simulink model "luenberger"  (Simulink 8.3)
settings: Solver=ode4  StartTime=0.0  StopTime=10.0  FixedStep=0.01  RelTol=1e-3
values from neighbouring files (symbols this model uses):
  A = [0 1 ... (first row only)    [por_model_obiekt_osX.m]    (also in wykresy.m)
  B = [0; k/omega0^2]    [por_model_obiekt_osX.m]    (also in wykresy.m)
  C = [1 0]    [por_model_obiekt_osX.m]    (also in wykresy.m)
  L = transpose(place(transpose(Al),transpose(Cl), [-1 -0.9 -1.1]))    [luenberger.m]
  X0 = [0 0]    [por_model_obiekt_osX.m]    (also in wykresy.m = [0.2738 0])
undefined symbols (not defined in the file or in its folder): A_, B_, C_
libraries: simulink x1
settings Model: Creator=student  LastModifiedBy=Maciek  CovSFcnEnable=on
settings OptimizationCC: ExpressionDepthLimit=2147483647
settings DebuggingCC: FcnCallInpInsideContextMsg=EnableAllAsWarning  FrameProcessingCompatibilityMsg=error
settings GRTTargetCC: CombineOutputUpdateFcns=on  GRTInterface=off

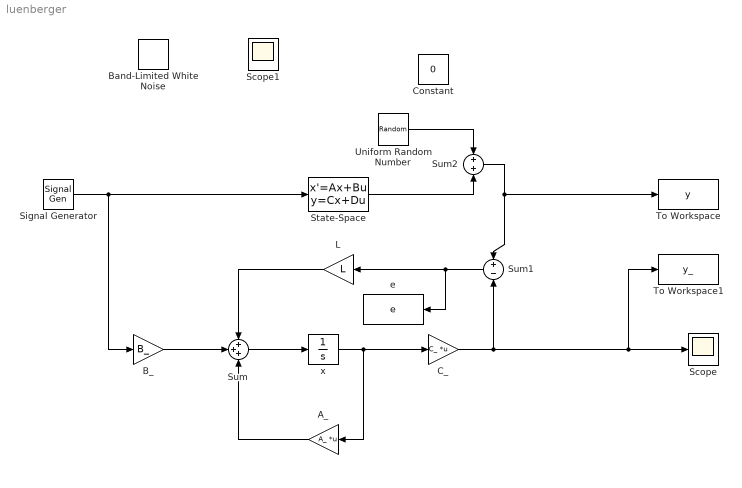
== system luenberger ==
  A_ : Gain  Gain=A_  Multiplication=Matrix(K*u) (u vector)
  B_ : Gain  Gain=B_
  Band-Limited White Noise : simulink/Sources/Band-Limited White Noise  Cov=[0.1]  Ts=0.1  seed=[23341]
  C_ : Gain  Gain=C_  Multiplication=Matrix(K*u) (u vector)
  Constant : Constant  Value=0
  L : Gain  Gain=L
  Scope : Scope
      settings: TimeRange=auto  LimitDataPoints=on  MaxDataPoints=5000  SaveToWorkspace=off  SaveName=ScopeData  YMin=-10  YMax=10  SampleTime=-1
  Scope1 : Scope
      settings: TimeRange=auto  LimitDataPoints=on  MaxDataPoints=5000  SaveToWorkspace=off  YMin=-1.00000  YMax=1.00000  SampleTime=-1
  Signal Generator : SignalGenerator
  State-Space : StateSpace  A=A  B=B  C=C  D=0  X0=X0
  Sum : Sum  Inputs=+++
  Sum1 : Sum  Inputs=+-
  Sum2 : Sum
  To Workspace : ToWorkspace  VariableName=y  SaveFormat=Timeseries  SampleTime=-1
  To Workspace1 : ToWorkspace  VariableName=y_  SaveFormat=Timeseries  SampleTime=-1
  Uniform Random Number : UniformRandomNumber  Minimum=-0.001  Maximum=0.001
  e : ToWorkspace  VariableName=e  SaveFormat=Timeseries  SampleTime=-1
  x : Integrator  InitialCondition=X0
  wires:
  Sum/1 -> x/1
  x/1 -> A_/1, C_/1
  A_/1 -> Sum/3
  C_/1 -> Sum1/2, Scope/1, To Workspace1/1
  Sum1/1 -> e/1, L/1
  L/1 -> Sum/1
  B_/1 -> Sum/2
  Signal Generator/1 -> State-Space/1, B_/1
  State-Space/1 -> Sum2/2
  Sum2/1 -> Sum1/1, To Workspace/1
  Uniform Random Number/1 -> Sum2/1
